simulink model "BumplessPID_UuT"  (R2020a)
settings: Solver=ode8  StartTime=0.0  StopTime=40  FixedStep=0.1  RelTol=1e-3
libraries: BumplessPID_Lib x1
settings Model: Creator=Christian  LastModifiedBy=Christian

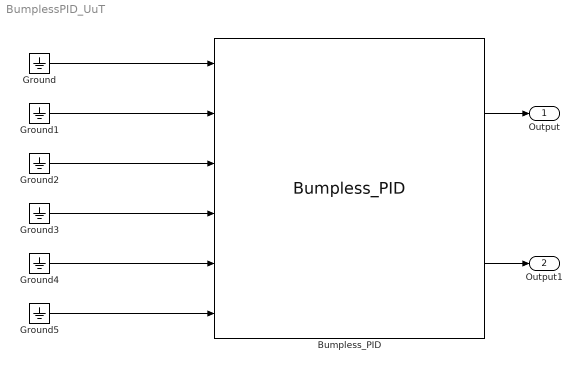
== system BumplessPID_UuT ==
  Bumpless_PID : BumplessPID_Lib/Bumpless_PID  SystemSampleTime=-1  Latency=0  AutoFrameSizeCalculation=off
  Ground{,1..5} (6 alike) : Ground
  Output : Outport
  Output1 : Outport  Port=2
  wires:
  Ground/1 -> Bumpless_PID/1
  Ground1/1 -> Bumpless_PID/2
  Ground2/1 -> Bumpless_PID/3
  Ground3/1 -> Bumpless_PID/4
  Ground4/1 -> Bumpless_PID/5
  Ground5/1 -> Bumpless_PID/6
  Bumpless_PID/1 -> Output/1
  Bumpless_PID/2 -> Output1/1
